simulink model "fusionAlg"  (R2018b)
settings: Solver=FixedStepDiscrete  StartTime=0.0  StopTime=inf  FixedStep=0.01  RelTol=1e-3
PostLoadFcn:
  | if any(exist('dsrtsu_mdlpostloadfcn', 'file') ~= 0), dsrtsu_mdlpostloadfcn('Execute', bdroot); end
model workspace (MAT data in the model file):
  handle : class17 (value not decoded)
(part 3 of 24)

== system fusionAlg/FUSION /FUS_DataAdapter/RadarAdapter/Subsystem42 ==
  <x6B_3B_Obj_27> : Inport
  Bus Creator : BusCreator  Inputs=2  OutDataTypeStr=Bus: FUS_UINT8_RESERVED_ST
      settings: InheritFromInputs=off
  Bus Creator1 : BusCreator  Inputs=17  OutDataTypeStr=Bus: FUS_RADAR_OBJ_ST  NonVirtualBus=on
      settings: InheritFromInputs=off
  Bus Selector1 : BusSelector  OutputSignals=Obj_ObstacleProb,Obj_XPos_Stdev,Obj_YPos_Stdev,Obj_XVelRel_Stdev,Obj_XAccRel,Obj_ExstProb,Obj_YVelRel,Obj_XVelRel,Obj_XPos,Obj_YPos,Obj_ID,Obj_UpdateFlag,Obj_ValidFlag,Obj_MotionPattern,Obj_Type,Obj_MeasFlag
  Constant : Constant  Value=0  OutDataTypeStr=uint8
  Constant1 : Constant  Value=0  OutDataTypeStr=uint8
  Data Type Conversion : DataTypeConversion  OutDataTypeStr=uint16
  Data Type Conversion{1..5} (5 alike) : DataTypeConversion  OutDataTypeStr=uint8
  <OBJ_27> : Outport
  wires:
  Bus Selector1/10 -> Bus Creator1/10  "<Obj_YPos>"
  Constant1/1 -> Bus Creator/2
  Bus Selector1/8 -> Bus Creator1/8  "<Obj_XVelRel>"
  Bus Selector1/14 -> Data Type Conversion3/1  "<Obj_MotionPattern>"
  Bus Creator1/1 -> <OBJ_27>/1
  Bus Selector1/11 -> Data Type Conversion/1  "<Obj_ID>"
  Bus Selector1/16 -> Data Type Conversion5/1  "<Obj_MeasFlag>"
  Bus Selector1/2 -> Bus Creator1/2  "<Obj_XPos_Stdev>"
  Bus Selector1/6 -> Bus Creator1/6  "<Obj_ExstProb>"
  Bus Selector1/1 -> Bus Creator1/1  "<Obj_ObstacleProb>"
  Bus Selector1/15 -> Data Type Conversion4/1  "<Obj_Type>"
  Constant/1 -> Bus Creator/1
  Bus Selector1/13 -> Data Type Conversion2/1  "<Obj_ValidFlag>"
  Bus Selector1/9 -> Bus Creator1/9  "<Obj_XPos>"
  Bus Selector1/4 -> Bus Creator1/4  "<Obj_XVelRel_Stdev>"
  Bus Selector1/3 -> Bus Creator1/3  "<Obj_YPos_Stdev>"
  Bus Selector1/5 -> Bus Creator1/5  "<Obj_XAccRel>"
  Bus Selector1/7 -> Bus Creator1/7  "<Obj_YVelRel>"
  Bus Selector1/12 -> Data Type Conversion1/1  "<Obj_UpdateFlag>"
  <x6B_3B_Obj_27>/1 -> Bus Selector1/1
  Bus Creator/1 -> Bus Creator1/17
  Data Type Conversion/1 -> Bus Creator1/11
  Data Type Conversion1/1 -> Bus Creator1/12
  Data Type Conversion2/1 -> Bus Creator1/13
  Data Type Conversion3/1 -> Bus Creator1/14
  Data Type Conversion4/1 -> Bus Creator1/15
  Data Type Conversion5/1 -> Bus Creator1/16

== system fusionAlg/FUSION /FUS_DataAdapter/RadarAdapter/Subsystem43 ==
  <x6C_3C_Obj_28> : Inport
  Bus Creator : BusCreator  Inputs=2  OutDataTypeStr=Bus: FUS_UINT8_RESERVED_ST
      settings: InheritFromInputs=off
  Bus Creator1 : BusCreator  Inputs=17  OutDataTypeStr=Bus: FUS_RADAR_OBJ_ST  NonVirtualBus=on
      settings: InheritFromInputs=off
  Bus Selector1 : BusSelector  OutputSignals=Obj_ObstacleProb,Obj_XPos_Stdev,Obj_YPos_Stdev,Obj_XVelRel_Stdev,Obj_XAccRel,Obj_ExstProb,Obj_YVelRel,Obj_XVelRel,Obj_XPos,Obj_YPos,Obj_ID,Obj_UpdateFlag,Obj_ValidFlag,Obj_MotionPattern,Obj_Type,Obj_MeasFlag
  Constant : Constant  Value=0  OutDataTypeStr=uint8
  Constant1 : Constant  Value=0  OutDataTypeStr=uint8
  Data Type Conversion : DataTypeConversion  OutDataTypeStr=uint16
  Data Type Conversion{1..5} (5 alike) : DataTypeConversion  OutDataTypeStr=uint8
  <OBJ_28> : Outport
  wires:
  Bus Selector1/10 -> Bus Creator1/10  "<Obj_YPos>"
  Constant1/1 -> Bus Creator/2
  Bus Selector1/8 -> Bus Creator1/8  "<Obj_XVelRel>"
  Bus Selector1/14 -> Data Type Conversion3/1  "<Obj_MotionPattern>"
  Bus Creator1/1 -> <OBJ_28>/1
  Bus Selector1/11 -> Data Type Conversion/1  "<Obj_ID>"
  Bus Selector1/16 -> Data Type Conversion5/1  "<Obj_MeasFlag>"
  Bus Selector1/2 -> Bus Creator1/2  "<Obj_XPos_Stdev>"
  Bus Selector1/6 -> Bus Creator1/6  "<Obj_ExstProb>"
  Bus Selector1/1 -> Bus Creator1/1  "<Obj_ObstacleProb>"
  Bus Selector1/15 -> Data Type Conversion4/1  "<Obj_Type>"
  Constant/1 -> Bus Creator/1
  Bus Selector1/13 -> Data Type Conversion2/1  "<Obj_ValidFlag>"
  Bus Selector1/9 -> Bus Creator1/9  "<Obj_XPos>"
  Bus Selector1/4 -> Bus Creator1/4  "<Obj_XVelRel_Stdev>"
  Bus Selector1/3 -> Bus Creator1/3  "<Obj_YPos_Stdev>"
  Bus Selector1/5 -> Bus Creator1/5  "<Obj_XAccRel>"
  Bus Selector1/7 -> Bus Creator1/7  "<Obj_YVelRel>"
  Bus Selector1/12 -> Data Type Conversion1/1  "<Obj_UpdateFlag>"
  <x6C_3C_Obj_28>/1 -> Bus Selector1/1
  Bus Creator/1 -> Bus Creator1/17
  Data Type Conversion/1 -> Bus Creator1/11
  Data Type Conversion1/1 -> Bus Creator1/12
  Data Type Conversion2/1 -> Bus Creator1/13
  Data Type Conversion3/1 -> Bus Creator1/14
  Data Type Conversion4/1 -> Bus Creator1/15
  Data Type Conversion5/1 -> Bus Creator1/16

== system fusionAlg/FUSION /FUS_DataAdapter/RadarAdapter/Subsystem44 ==
  <x6D_3D_Obj_29> : Inport
  Bus Creator : BusCreator  Inputs=2  OutDataTypeStr=Bus: FUS_UINT8_RESERVED_ST
      settings: InheritFromInputs=off
  Bus Creator1 : BusCreator  Inputs=17  OutDataTypeStr=Bus: FUS_RADAR_OBJ_ST  NonVirtualBus=on
      settings: InheritFromInputs=off
  Bus Selector1 : BusSelector  OutputSignals=Obj_ObstacleProb,Obj_XPos_Stdev,Obj_YPos_Stdev,Obj_XVelRel_Stdev,Obj_XAccRel,Obj_ExstProb,Obj_YVelRel,Obj_XVelRel,Obj_XPos,Obj_YPos,Obj_ID,Obj_UpdateFlag,Obj_ValidFlag,Obj_MotionPattern,Obj_Type,Obj_MeasFlag
  Constant : Constant  Value=0  OutDataTypeStr=uint8
  Constant1 : Constant  Value=0  OutDataTypeStr=uint8
  Data Type Conversion : DataTypeConversion  OutDataTypeStr=uint16
  Data Type Conversion{1..5} (5 alike) : DataTypeConversion  OutDataTypeStr=uint8
  <OBJ_29> : Outport
  wires:
  Bus Selector1/10 -> Bus Creator1/10  "<Obj_YPos>"
  Constant1/1 -> Bus Creator/2
  Bus Selector1/8 -> Bus Creator1/8  "<Obj_XVelRel>"
  Bus Selector1/14 -> Data Type Conversion3/1  "<Obj_MotionPattern>"
  Bus Creator1/1 -> <OBJ_29>/1
  Bus Selector1/11 -> Data Type Conversion/1  "<Obj_ID>"
  Bus Selector1/16 -> Data Type Conversion5/1  "<Obj_MeasFlag>"
  Bus Selector1/2 -> Bus Creator1/2  "<Obj_XPos_Stdev>"
  Bus Selector1/6 -> Bus Creator1/6  "<Obj_ExstProb>"
  Bus Selector1/1 -> Bus Creator1/1  "<Obj_ObstacleProb>"
  Bus Selector1/15 -> Data Type Conversion4/1  "<Obj_Type>"
  Constant/1 -> Bus Creator/1
  Bus Selector1/13 -> Data Type Conversion2/1  "<Obj_ValidFlag>"
  Bus Selector1/9 -> Bus Creator1/9  "<Obj_XPos>"
  Bus Selector1/4 -> Bus Creator1/4  "<Obj_XVelRel_Stdev>"
  Bus Selector1/3 -> Bus Creator1/3  "<Obj_YPos_Stdev>"
  Bus Selector1/5 -> Bus Creator1/5  "<Obj_XAccRel>"
  Bus Selector1/7 -> Bus Creator1/7  "<Obj_YVelRel>"
  Bus Selector1/12 -> Data Type Conversion1/1  "<Obj_UpdateFlag>"
  <x6D_3D_Obj_29>/1 -> Bus Selector1/1
  Bus Creator/1 -> Bus Creator1/17
  Data Type Conversion/1 -> Bus Creator1/11
  Data Type Conversion1/1 -> Bus Creator1/12
  Data Type Conversion2/1 -> Bus Creator1/13
  Data Type Conversion3/1 -> Bus Creator1/14
  Data Type Conversion4/1 -> Bus Creator1/15
  Data Type Conversion5/1 -> Bus Creator1/16

== system fusionAlg/FUSION /FUS_DataAdapter/RadarAdapter/Subsystem45 ==
  <x6E_3E_Obj_30> : Inport
  Bus Creator : BusCreator  Inputs=2  OutDataTypeStr=Bus: FUS_UINT8_RESERVED_ST
      settings: InheritFromInputs=off
  Bus Creator1 : BusCreator  Inputs=17  OutDataTypeStr=Bus: FUS_RADAR_OBJ_ST  NonVirtualBus=on
      settings: InheritFromInputs=off
  Bus Selector1 : BusSelector  OutputSignals=Obj_ObstacleProb,Obj_XPos_Stdev,Obj_YPos_Stdev,Obj_XVelRel_Stdev,Obj_XAccRel,Obj_ExstProb,Obj_YVelRel,Obj_XVelRel,Obj_XPos,Obj_YPos,Obj_ID,Obj_UpdateFlag,Obj_ValidFlag,Obj_MotionPattern,Obj_Type,Obj_MeasFlag
  Constant : Constant  Value=0  OutDataTypeStr=uint8
  Constant1 : Constant  Value=0  OutDataTypeStr=uint8
  Data Type Conversion : DataTypeConversion  OutDataTypeStr=uint16
  Data Type Conversion{1..5} (5 alike) : DataTypeConversion  OutDataTypeStr=uint8
  <OBJ_30> : Outport
  wires:
  Bus Selector1/10 -> Bus Creator1/10  "<Obj_YPos>"
  Constant1/1 -> Bus Creator/2
  Bus Selector1/8 -> Bus Creator1/8  "<Obj_XVelRel>"
  Bus Selector1/14 -> Data Type Conversion3/1  "<Obj_MotionPattern>"
  Bus Creator1/1 -> <OBJ_30>/1
  Bus Selector1/11 -> Data Type Conversion/1  "<Obj_ID>"
  Bus Selector1/16 -> Data Type Conversion5/1  "<Obj_MeasFlag>"
  Bus Selector1/2 -> Bus Creator1/2  "<Obj_XPos_Stdev>"
  Bus Selector1/6 -> Bus Creator1/6  "<Obj_ExstProb>"
  Bus Selector1/1 -> Bus Creator1/1  "<Obj_ObstacleProb>"
  Bus Selector1/15 -> Data Type Conversion4/1  "<Obj_Type>"
  Constant/1 -> Bus Creator/1
  Bus Selector1/13 -> Data Type Conversion2/1  "<Obj_ValidFlag>"
  Bus Selector1/9 -> Bus Creator1/9  "<Obj_XPos>"
  Bus Selector1/4 -> Bus Creator1/4  "<Obj_XVelRel_Stdev>"
  Bus Selector1/3 -> Bus Creator1/3  "<Obj_YPos_Stdev>"
  Bus Selector1/5 -> Bus Creator1/5  "<Obj_XAccRel>"
  Bus Selector1/7 -> Bus Creator1/7  "<Obj_YVelRel>"
  Bus Selector1/12 -> Data Type Conversion1/1  "<Obj_UpdateFlag>"
  <x6E_3E_Obj_30>/1 -> Bus Selector1/1
  Bus Creator/1 -> Bus Creator1/17
  Data Type Conversion/1 -> Bus Creator1/11
  Data Type Conversion1/1 -> Bus Creator1/12
  Data Type Conversion2/1 -> Bus Creator1/13
  Data Type Conversion3/1 -> Bus Creator1/14
  Data Type Conversion4/1 -> Bus Creator1/15
  Data Type Conversion5/1 -> Bus Creator1/16

== system fusionAlg/FUSION /FUS_DataAdapter/RadarAdapter/Subsystem46 ==
  <x6F_3F_Obj_31> : Inport
  Bus Creator : BusCreator  Inputs=2  OutDataTypeStr=Bus: FUS_UINT8_RESERVED_ST
      settings: InheritFromInputs=off
  Bus Creator1 : BusCreator  Inputs=17  OutDataTypeStr=Bus: FUS_RADAR_OBJ_ST  NonVirtualBus=on
      settings: InheritFromInputs=off
  Bus Selector1 : BusSelector  OutputSignals=Obj_ObstacleProb,Obj_XPos_Stdev,Obj_YPos_Stdev,Obj_XVelRel_Stdev,Obj_XAccRel,Obj_ExstProb,Obj_YVelRel,Obj_XVelRel,Obj_XPos,Obj_YPos,Obj_ID,Obj_UpdateFlag,Obj_ValidFlag,Obj_MotionPattern,Obj_Type,Obj_MeasFlag
  Constant : Constant  Value=0  OutDataTypeStr=uint8
  Constant1 : Constant  Value=0  OutDataTypeStr=uint8
  Data Type Conversion : DataTypeConversion  OutDataTypeStr=uint16
  Data Type Conversion{1..5} (5 alike) : DataTypeConversion  OutDataTypeStr=uint8
  <OBJ_31> : Outport
  wires:
  Bus Selector1/10 -> Bus Creator1/10  "<Obj_YPos>"
  Constant1/1 -> Bus Creator/2
  Bus Selector1/8 -> Bus Creator1/8  "<Obj_XVelRel>"
  Bus Selector1/14 -> Data Type Conversion3/1  "<Obj_MotionPattern>"
  Bus Creator1/1 -> <OBJ_31>/1
  Bus Selector1/11 -> Data Type Conversion/1  "<Obj_ID>"
  Bus Selector1/16 -> Data Type Conversion5/1  "<Obj_MeasFlag>"
  Bus Selector1/2 -> Bus Creator1/2  "<Obj_XPos_Stdev>"
  Bus Selector1/6 -> Bus Creator1/6  "<Obj_ExstProb>"
  Bus Selector1/1 -> Bus Creator1/1  "<Obj_ObstacleProb>"
  Bus Selector1/15 -> Data Type Conversion4/1  "<Obj_Type>"
  Constant/1 -> Bus Creator/1
  Bus Selector1/13 -> Data Type Conversion2/1  "<Obj_ValidFlag>"
  Bus Selector1/9 -> Bus Creator1/9  "<Obj_XPos>"
  Bus Selector1/4 -> Bus Creator1/4  "<Obj_XVelRel_Stdev>"
  Bus Selector1/3 -> Bus Creator1/3  "<Obj_YPos_Stdev>"
  Bus Selector1/5 -> Bus Creator1/5  "<Obj_XAccRel>"
  Bus Selector1/7 -> Bus Creator1/7  "<Obj_YVelRel>"
  Bus Selector1/12 -> Data Type Conversion1/1  "<Obj_UpdateFlag>"
  <x6F_3F_Obj_31>/1 -> Bus Selector1/1
  Bus Creator/1 -> Bus Creator1/17
  Data Type Conversion/1 -> Bus Creator1/11
  Data Type Conversion1/1 -> Bus Creator1/12
  Data Type Conversion2/1 -> Bus Creator1/13
  Data Type Conversion3/1 -> Bus Creator1/14
  Data Type Conversion4/1 -> Bus Creator1/15
  Data Type Conversion5/1 -> Bus Creator1/16

== system fusionAlg/FUSION /FUS_DataAdapter/RadarAdapter/Subsystem47 ==
  <x70_40_Obj_32> : Inport
  Bus Creator : BusCreator  Inputs=2  OutDataTypeStr=Bus: FUS_UINT8_RESERVED_ST
      settings: InheritFromInputs=off
  Bus Creator1 : BusCreator  Inputs=17  OutDataTypeStr=Bus: FUS_RADAR_OBJ_ST  NonVirtualBus=on
      settings: InheritFromInputs=off
  Bus Selector1 : BusSelector  OutputSignals=Obj_ObstacleProb,Obj_XPos_Stdev,Obj_YPos_Stdev,Obj_XVelRel_Stdev,Obj_XAccRel,Obj_ExstProb,Obj_YVelRel,Obj_XVelRel,Obj_XPos,Obj_YPos,Obj_ID,Obj_UpdateFlag,Obj_ValidFlag,Obj_MotionPattern,Obj_Type,Obj_MeasFlag
  Constant : Constant  Value=0  OutDataTypeStr=uint8
  Constant1 : Constant  Value=0  OutDataTypeStr=uint8
  Data Type Conversion : DataTypeConversion  OutDataTypeStr=uint16
  Data Type Conversion{1..5} (5 alike) : DataTypeConversion  OutDataTypeStr=uint8
  <OBJ_32> : Outport
  wires:
  Bus Selector1/10 -> Bus Creator1/10  "<Obj_YPos>"
  Constant1/1 -> Bus Creator/2
  Bus Selector1/8 -> Bus Creator1/8  "<Obj_XVelRel>"
  Bus Selector1/14 -> Data Type Conversion3/1  "<Obj_MotionPattern>"
  Bus Creator1/1 -> <OBJ_32>/1
  Bus Selector1/11 -> Data Type Conversion/1  "<Obj_ID>"
  Bus Selector1/16 -> Data Type Conversion5/1  "<Obj_MeasFlag>"
  Bus Selector1/2 -> Bus Creator1/2  "<Obj_XPos_Stdev>"
  Bus Selector1/6 -> Bus Creator1/6  "<Obj_ExstProb>"
  Bus Selector1/1 -> Bus Creator1/1  "<Obj_ObstacleProb>"
  Bus Selector1/15 -> Data Type Conversion4/1  "<Obj_Type>"
  Constant/1 -> Bus Creator/1
  Bus Selector1/13 -> Data Type Conversion2/1  "<Obj_ValidFlag>"
  Bus Selector1/9 -> Bus Creator1/9  "<Obj_XPos>"
  Bus Selector1/4 -> Bus Creator1/4  "<Obj_XVelRel_Stdev>"
  Bus Selector1/3 -> Bus Creator1/3  "<Obj_YPos_Stdev>"
  Bus Selector1/5 -> Bus Creator1/5  "<Obj_XAccRel>"
  Bus Selector1/7 -> Bus Creator1/7  "<Obj_YVelRel>"
  Bus Selector1/12 -> Data Type Conversion1/1  "<Obj_UpdateFlag>"
  <x70_40_Obj_32>/1 -> Bus Selector1/1
  Bus Creator/1 -> Bus Creator1/17
  Data Type Conversion/1 -> Bus Creator1/11
  Data Type Conversion1/1 -> Bus Creator1/12
  Data Type Conversion2/1 -> Bus Creator1/13
  Data Type Conversion3/1 -> Bus Creator1/14
  Data Type Conversion4/1 -> Bus Creator1/15
  Data Type Conversion5/1 -> Bus Creator1/16

== system fusionAlg/FUSION /FUS_DataAdapter/RadarAdapter/Subsystem48 ==
  <x71_41_Obj_33> : Inport
  Bus Creator : BusCreator  Inputs=2  OutDataTypeStr=Bus: FUS_UINT8_RESERVED_ST
      settings: InheritFromInputs=off
  Bus Creator1 : BusCreator  Inputs=17  OutDataTypeStr=Bus: FUS_RADAR_OBJ_ST  NonVirtualBus=on
      settings: InheritFromInputs=off
  Bus Selector1 : BusSelector  OutputSignals=Obj_ObstacleProb,Obj_XPos_Stdev,Obj_YPos_Stdev,Obj_XVelRel_Stdev,Obj_XAccRel,Obj_ExstProb,Obj_YVelRel,Obj_XVelRel,Obj_XPos,Obj_YPos,Obj_ID,Obj_UpdateFlag,Obj_ValidFlag,Obj_MotionPattern,Obj_Type,Obj_MeasFlag
  Constant : Constant  Value=0  OutDataTypeStr=uint8
  Constant1 : Constant  Value=0  OutDataTypeStr=uint8
  Data Type Conversion : DataTypeConversion  OutDataTypeStr=uint16
  Data Type Conversion{1..5} (5 alike) : DataTypeConversion  OutDataTypeStr=uint8
  <OBJ_33> : Outport
  wires:
  Bus Selector1/10 -> Bus Creator1/10  "<Obj_YPos>"
  Constant1/1 -> Bus Creator/2
  Bus Selector1/8 -> Bus Creator1/8  "<Obj_XVelRel>"
  Bus Selector1/14 -> Data Type Conversion3/1  "<Obj_MotionPattern>"
  Bus Creator1/1 -> <OBJ_33>/1
  Bus Selector1/11 -> Data Type Conversion/1  "<Obj_ID>"
  Bus Selector1/16 -> Data Type Conversion5/1  "<Obj_MeasFlag>"
  Bus Selector1/2 -> Bus Creator1/2  "<Obj_XPos_Stdev>"
  Bus Selector1/6 -> Bus Creator1/6  "<Obj_ExstProb>"
  Bus Selector1/1 -> Bus Creator1/1  "<Obj_ObstacleProb>"
  Bus Selector1/15 -> Data Type Conversion4/1  "<Obj_Type>"
  Constant/1 -> Bus Creator/1
  Bus Selector1/13 -> Data Type Conversion2/1  "<Obj_ValidFlag>"
  Bus Selector1/9 -> Bus Creator1/9  "<Obj_XPos>"
  Bus Selector1/4 -> Bus Creator1/4  "<Obj_XVelRel_Stdev>"
  Bus Selector1/3 -> Bus Creator1/3  "<Obj_YPos_Stdev>"
  Bus Selector1/5 -> Bus Creator1/5  "<Obj_XAccRel>"
  Bus Selector1/7 -> Bus Creator1/7  "<Obj_YVelRel>"
  Bus Selector1/12 -> Data Type Conversion1/1  "<Obj_UpdateFlag>"
  <x71_41_Obj_33>/1 -> Bus Selector1/1
  Bus Creator/1 -> Bus Creator1/17
  Data Type Conversion/1 -> Bus Creator1/11
  Data Type Conversion1/1 -> Bus Creator1/12
  Data Type Conversion2/1 -> Bus Creator1/13
  Data Type Conversion3/1 -> Bus Creator1/14
  Data Type Conversion4/1 -> Bus Creator1/15
  Data Type Conversion5/1 -> Bus Creator1/16

== system fusionAlg/FUSION /FUS_DataAdapter/RadarAdapter/Subsystem5 ==
  <x55_25_Obj_05> : Inport
  Bus Creator : BusCreator  Inputs=2  OutDataTypeStr=Bus: FUS_UINT8_RESERVED_ST
      settings: InheritFromInputs=off
  Bus Creator1 : BusCreator  Inputs=17  OutDataTypeStr=Bus: FUS_RADAR_OBJ_ST  NonVirtualBus=on
      settings: InheritFromInputs=off
  Bus Selector1 : BusSelector  OutputSignals=Obj_ObstacleProb,Obj_XPos_Stdev,Obj_YPos_Stdev,Obj_XVelRel_Stdev,Obj_XAccRel,Obj_ExstProb,Obj_YVelRel,Obj_XVelRel,Obj_XPos,Obj_YPos,Obj_ID,Obj_UpdateFlag,Obj_ValidFlag,Obj_MotionPattern,Obj_Type,Obj_MeasFlag
  Constant : Constant  Value=0  OutDataTypeStr=uint8
  Constant1 : Constant  Value=0  OutDataTypeStr=uint8
  Data Type Conversion : DataTypeConversion  OutDataTypeStr=uint16
  Data Type Conversion{1..5} (5 alike) : DataTypeConversion  OutDataTypeStr=uint8
  <OBJ_05> : Outport
  wires:
  Bus Selector1/10 -> Bus Creator1/10  "<Obj_YPos>"
  Constant1/1 -> Bus Creator/2
  Bus Selector1/8 -> Bus Creator1/8  "<Obj_XVelRel>"
  Bus Selector1/14 -> Data Type Conversion3/1  "<Obj_MotionPattern>"
  Bus Creator1/1 -> <OBJ_05>/1
  Bus Selector1/11 -> Data Type Conversion/1  "<Obj_ID>"
  Bus Selector1/16 -> Data Type Conversion5/1  "<Obj_MeasFlag>"
  Bus Selector1/2 -> Bus Creator1/2  "<Obj_XPos_Stdev>"
  Bus Selector1/6 -> Bus Creator1/6  "<Obj_ExstProb>"
  Bus Selector1/1 -> Bus Creator1/1  "<Obj_ObstacleProb>"
  Bus Selector1/15 -> Data Type Conversion4/1  "<Obj_Type>"
  Constant/1 -> Bus Creator/1
  Bus Selector1/13 -> Data Type Conversion2/1  "<Obj_ValidFlag>"
  Bus Selector1/9 -> Bus Creator1/9  "<Obj_XPos>"
  Bus Selector1/4 -> Bus Creator1/4  "<Obj_XVelRel_Stdev>"
  Bus Selector1/3 -> Bus Creator1/3  "<Obj_YPos_Stdev>"
  Bus Selector1/5 -> Bus Creator1/5  "<Obj_XAccRel>"
  Bus Selector1/7 -> Bus Creator1/7  "<Obj_YVelRel>"
  Bus Selector1/12 -> Data Type Conversion1/1  "<Obj_UpdateFlag>"
  <x55_25_Obj_05>/1 -> Bus Selector1/1
  Bus Creator/1 -> Bus Creator1/17
  Data Type Conversion/1 -> Bus Creator1/11
  Data Type Conversion1/1 -> Bus Creator1/12
  Data Type Conversion2/1 -> Bus Creator1/13
  Data Type Conversion3/1 -> Bus Creator1/14
  Data Type Conversion4/1 -> Bus Creator1/15
  Data Type Conversion5/1 -> Bus Creator1/16

== system fusionAlg/FUSION /FUS_DataAdapter/RadarAdapter/Subsystem6 ==
  <x56_26_Obj_06> : Inport
  Bus Creator : BusCreator  Inputs=2  OutDataTypeStr=Bus: FUS_UINT8_RESERVED_ST
      settings: InheritFromInputs=off
  Bus Creator1 : BusCreator  Inputs=17  OutDataTypeStr=Bus: FUS_RADAR_OBJ_ST  NonVirtualBus=on
      settings: InheritFromInputs=off
  Bus Selector1 : BusSelector  OutputSignals=Obj_ObstacleProb,Obj_XPos_Stdev,Obj_YPos_Stdev,Obj_XVelRel_Stdev,Obj_XAccRel,Obj_ExstProb,Obj_YVelRel,Obj_XVelRel,Obj_XPos,Obj_YPos,Obj_ID,Obj_UpdateFlag,Obj_ValidFlag,Obj_MotionPattern,Obj_Type,Obj_MeasFlag
  Constant : Constant  Value=0  OutDataTypeStr=uint8
  Constant1 : Constant  Value=0  OutDataTypeStr=uint8
  Data Type Conversion : DataTypeConversion  OutDataTypeStr=uint16
  Data Type Conversion{1..5} (5 alike) : DataTypeConversion  OutDataTypeStr=uint8
  <OBJ_06> : Outport
  wires:
  Bus Selector1/10 -> Bus Creator1/10  "<Obj_YPos>"
  Constant1/1 -> Bus Creator/2
  Bus Selector1/8 -> Bus Creator1/8  "<Obj_XVelRel>"
  Bus Selector1/14 -> Data Type Conversion3/1  "<Obj_MotionPattern>"
  Bus Creator1/1 -> <OBJ_06>/1
  Bus Selector1/11 -> Data Type Conversion/1  "<Obj_ID>"
  Bus Selector1/16 -> Data Type Conversion5/1  "<Obj_MeasFlag>"
  Bus Selector1/2 -> Bus Creator1/2  "<Obj_XPos_Stdev>"
  Bus Selector1/6 -> Bus Creator1/6  "<Obj_ExstProb>"
  Bus Selector1/1 -> Bus Creator1/1  "<Obj_ObstacleProb>"
  Bus Selector1/15 -> Data Type Conversion4/1  "<Obj_Type>"
  Constant/1 -> Bus Creator/1
  Bus Selector1/13 -> Data Type Conversion2/1  "<Obj_ValidFlag>"
  Bus Selector1/9 -> Bus Creator1/9  "<Obj_XPos>"
  Bus Selector1/4 -> Bus Creator1/4  "<Obj_XVelRel_Stdev>"
  Bus Selector1/3 -> Bus Creator1/3  "<Obj_YPos_Stdev>"
  Bus Selector1/5 -> Bus Creator1/5  "<Obj_XAccRel>"
  Bus Selector1/7 -> Bus Creator1/7  "<Obj_YVelRel>"
  Bus Selector1/12 -> Data Type Conversion1/1  "<Obj_UpdateFlag>"
  <x56_26_Obj_06>/1 -> Bus Selector1/1
  Bus Creator/1 -> Bus Creator1/17
  Data Type Conversion/1 -> Bus Creator1/11
  Data Type Conversion1/1 -> Bus Creator1/12
  Data Type Conversion2/1 -> Bus Creator1/13
  Data Type Conversion3/1 -> Bus Creator1/14
  Data Type Conversion4/1 -> Bus Creator1/15
  Data Type Conversion5/1 -> Bus Creator1/16

== system fusionAlg/FUSION /FUS_DataAdapter/RadarAdapter/Subsystem7 ==
  <x57_27_Obj_07> : Inport
  Bus Creator : BusCreator  Inputs=2  OutDataTypeStr=Bus: FUS_UINT8_RESERVED_ST
      settings: InheritFromInputs=off
  Bus Creator1 : BusCreator  Inputs=17  OutDataTypeStr=Bus: FUS_RADAR_OBJ_ST  NonVirtualBus=on
      settings: InheritFromInputs=off
  Bus Selector1 : BusSelector  OutputSignals=Obj_ObstacleProb,Obj_XPos_Stdev,Obj_YPos_Stdev,Obj_XVelRel_Stdev,Obj_XAccRel,Obj_ExstProb,Obj_YVelRel,Obj_XVelRel,Obj_XPos,Obj_YPos,Obj_ID,Obj_UpdateFlag,Obj_ValidFlag,Obj_MotionPattern,Obj_Type,Obj_MeasFlag
  Constant : Constant  Value=0  OutDataTypeStr=uint8
  Constant1 : Constant  Value=0  OutDataTypeStr=uint8
  Data Type Conversion : DataTypeConversion  OutDataTypeStr=uint16
  Data Type Conversion{1..5} (5 alike) : DataTypeConversion  OutDataTypeStr=uint8
  <OBJ_07> : Outport
  wires:
  Bus Selector1/10 -> Bus Creator1/10  "<Obj_YPos>"
  Constant1/1 -> Bus Creator/2
  Bus Selector1/8 -> Bus Creator1/8  "<Obj_XVelRel>"
  Bus Selector1/14 -> Data Type Conversion3/1  "<Obj_MotionPattern>"
  Bus Creator1/1 -> <OBJ_07>/1
  Bus Selector1/11 -> Data Type Conversion/1  "<Obj_ID>"
  Bus Selector1/16 -> Data Type Conversion5/1  "<Obj_MeasFlag>"
  Bus Selector1/2 -> Bus Creator1/2  "<Obj_XPos_Stdev>"
  Bus Selector1/6 -> Bus Creator1/6  "<Obj_ExstProb>"
  Bus Selector1/1 -> Bus Creator1/1  "<Obj_ObstacleProb>"
  Bus Selector1/15 -> Data Type Conversion4/1  "<Obj_Type>"
  Constant/1 -> Bus Creator/1
  Bus Selector1/13 -> Data Type Conversion2/1  "<Obj_ValidFlag>"
  Bus Selector1/9 -> Bus Creator1/9  "<Obj_XPos>"
  Bus Selector1/4 -> Bus Creator1/4  "<Obj_XVelRel_Stdev>"
  Bus Selector1/3 -> Bus Creator1/3  "<Obj_YPos_Stdev>"
  Bus Selector1/5 -> Bus Creator1/5  "<Obj_XAccRel>"
  Bus Selector1/7 -> Bus Creator1/7  "<Obj_YVelRel>"
  Bus Selector1/12 -> Data Type Conversion1/1  "<Obj_UpdateFlag>"
  <x57_27_Obj_07>/1 -> Bus Selector1/1
  Bus Creator/1 -> Bus Creator1/17
  Data Type Conversion/1 -> Bus Creator1/11
  Data Type Conversion1/1 -> Bus Creator1/12
  Data Type Conversion2/1 -> Bus Creator1/13
  Data Type Conversion3/1 -> Bus Creator1/14
  Data Type Conversion4/1 -> Bus Creator1/15
  Data Type Conversion5/1 -> Bus Creator1/16

== system fusionAlg/FUSION /FUS_DataAdapter/RadarAdapter/Subsystem8 ==
  <x58_28_Obj_08> : Inport
  Bus Creator : BusCreator  Inputs=2  OutDataTypeStr=Bus: FUS_UINT8_RESERVED_ST
      settings: InheritFromInputs=off
  Bus Creator1 : BusCreator  Inputs=17  OutDataTypeStr=Bus: FUS_RADAR_OBJ_ST  NonVirtualBus=on
      settings: InheritFromInputs=off
  Bus Selector1 : BusSelector  OutputSignals=Obj_ObstacleProb,Obj_XPos_Stdev,Obj_YPos_Stdev,Obj_XVelRel_Stdev,Obj_XAccRel,Obj_ExstProb,Obj_YVelRel,Obj_XVelRel,Obj_XPos,Obj_YPos,Obj_ID,Obj_UpdateFlag,Obj_ValidFlag,Obj_MotionPattern,Obj_Type,Obj_MeasFlag
  Constant : Constant  Value=0  OutDataTypeStr=uint8
  Constant1 : Constant  Value=0  OutDataTypeStr=uint8
  Data Type Conversion : DataTypeConversion  OutDataTypeStr=uint16
  Data Type Conversion{1..5} (5 alike) : DataTypeConversion  OutDataTypeStr=uint8
  <OBJ_08> : Outport
  wires:
  Bus Selector1/10 -> Bus Creator1/10  "<Obj_YPos>"
  Constant1/1 -> Bus Creator/2
  Bus Selector1/8 -> Bus Creator1/8  "<Obj_XVelRel>"
  Bus Selector1/14 -> Data Type Conversion3/1  "<Obj_MotionPattern>"
  Bus Creator1/1 -> <OBJ_08>/1
  Bus Selector1/11 -> Data Type Conversion/1  "<Obj_ID>"
  Bus Selector1/16 -> Data Type Conversion5/1  "<Obj_MeasFlag>"
  Bus Selector1/2 -> Bus Creator1/2  "<Obj_XPos_Stdev>"
  Bus Selector1/6 -> Bus Creator1/6  "<Obj_ExstProb>"
  Bus Selector1/1 -> Bus Creator1/1  "<Obj_ObstacleProb>"
  Bus Selector1/15 -> Data Type Conversion4/1  "<Obj_Type>"
  Constant/1 -> Bus Creator/1
  Bus Selector1/13 -> Data Type Conversion2/1  "<Obj_ValidFlag>"
  Bus Selector1/9 -> Bus Creator1/9  "<Obj_XPos>"
  Bus Selector1/4 -> Bus Creator1/4  "<Obj_XVelRel_Stdev>"
  Bus Selector1/3 -> Bus Creator1/3  "<Obj_YPos_Stdev>"
  Bus Selector1/5 -> Bus Creator1/5  "<Obj_XAccRel>"
  Bus Selector1/7 -> Bus Creator1/7  "<Obj_YVelRel>"
  Bus Selector1/12 -> Data Type Conversion1/1  "<Obj_UpdateFlag>"
  <x58_28_Obj_08>/1 -> Bus Selector1/1
  Bus Creator/1 -> Bus Creator1/17
  Data Type Conversion/1 -> Bus Creator1/11
  Data Type Conversion1/1 -> Bus Creator1/12
  Data Type Conversion2/1 -> Bus Creator1/13
  Data Type Conversion3/1 -> Bus Creator1/14
  Data Type Conversion4/1 -> Bus Creator1/15
  Data Type Conversion5/1 -> Bus Creator1/16

== system fusionAlg/FUSION /FUS_DataAdapter/RadarAdapter/Subsystem9 ==
  <x59_29_Obj_09> : Inport
  Bus Creator : BusCreator  Inputs=2  OutDataTypeStr=Bus: FUS_UINT8_RESERVED_ST
      settings: InheritFromInputs=off
  Bus Creator1 : BusCreator  Inputs=17  OutDataTypeStr=Bus: FUS_RADAR_OBJ_ST  NonVirtualBus=on
      settings: InheritFromInputs=off
  Bus Selector1 : BusSelector  OutputSignals=Obj_ObstacleProb,Obj_XPos_Stdev,Obj_YPos_Stdev,Obj_XVelRel_Stdev,Obj_XAccRel,Obj_ExstProb,Obj_YVelRel,Obj_XVelRel,Obj_XPos,Obj_YPos,Obj_ID,Obj_UpdateFlag,Obj_ValidFlag,Obj_MotionPattern,Obj_Type,Obj_MeasFlag
  Constant : Constant  Value=0  OutDataTypeStr=uint8
  Constant1 : Constant  Value=0  OutDataTypeStr=uint8
  Data Type Conversion : DataTypeConversion  OutDataTypeStr=uint16
  Data Type Conversion{1..5} (5 alike) : DataTypeConversion  OutDataTypeStr=uint8
  <OBJ_09> : Outport
  wires:
  Bus Selector1/10 -> Bus Creator1/10  "<Obj_YPos>"
  Constant1/1 -> Bus Creator/2
  Bus Selector1/8 -> Bus Creator1/8  "<Obj_XVelRel>"
  Bus Selector1/14 -> Data Type Conversion3/1  "<Obj_MotionPattern>"
  Bus Creator1/1 -> <OBJ_09>/1
  Bus Selector1/11 -> Data Type Conversion/1  "<Obj_ID>"
  Bus Selector1/16 -> Data Type Conversion5/1  "<Obj_MeasFlag>"
  Bus Selector1/2 -> Bus Creator1/2  "<Obj_XPos_Stdev>"
  Bus Selector1/6 -> Bus Creator1/6  "<Obj_ExstProb>"
  Bus Selector1/1 -> Bus Creator1/1  "<Obj_ObstacleProb>"
  Bus Selector1/15 -> Data Type Conversion4/1  "<Obj_Type>"
  Constant/1 -> Bus Creator/1
  Bus Selector1/13 -> Data Type Conversion2/1  "<Obj_ValidFlag>"
  Bus Selector1/9 -> Bus Creator1/9  "<Obj_XPos>"
  Bus Selector1/4 -> Bus Creator1/4  "<Obj_XVelRel_Stdev>"
  Bus Selector1/3 -> Bus Creator1/3  "<Obj_YPos_Stdev>"
  Bus Selector1/5 -> Bus Creator1/5  "<Obj_XAccRel>"
  Bus Selector1/7 -> Bus Creator1/7  "<Obj_YVelRel>"
  Bus Selector1/12 -> Data Type Conversion1/1  "<Obj_UpdateFlag>"
  <x59_29_Obj_09>/1 -> Bus Selector1/1
  Bus Creator/1 -> Bus Creator1/17
  Data Type Conversion/1 -> Bus Creator1/11
  Data Type Conversion1/1 -> Bus Creator1/12
  Data Type Conversion2/1 -> Bus Creator1/13
  Data Type Conversion3/1 -> Bus Creator1/14
  Data Type Conversion4/1 -> Bus Creator1/15
  Data Type Conversion5/1 -> Bus Creator1/16

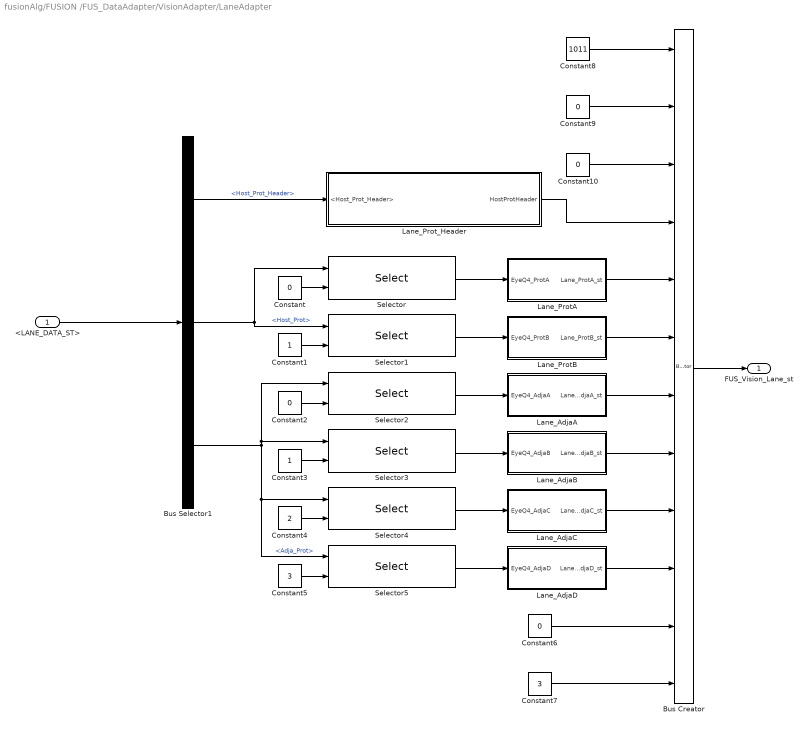
== system fusionAlg/FUSION /FUS_DataAdapter/VisionAdapter/LaneAdapter ==
  <LANE_DATA_ST> : Inport
  Bus Creator : BusCreator  Inputs=12  OutDataTypeStr=Bus: FUS_EYEQ4_LANE_DATA_ST  NonVirtualBus=on
      settings: InheritFromInputs=off
  Bus Selector1 : BusSelector  OutputSignals=Host_Prot_Header,Host_Prot,Adja_Prot
  Constant : Constant  Value=0  OutDataTypeStr=uint8
  Constant1 : Constant  OutDataTypeStr=uint8
  Constant10 : Constant  Value=0  OutDataTypeStr=uint32
  Constant2 : Constant  Value=0  OutDataTypeStr=uint8
  Constant3 : Constant  OutDataTypeStr=uint8
  Constant4 : Constant  Value=2  OutDataTypeStr=uint8
  Constant5 : Constant  Value=3  OutDataTypeStr=uint8
  Constant6 : Constant  Value=0  OutDataTypeStr=uint32
  Constant7 : Constant  Value=3  OutDataTypeStr=uint32
  Constant8 : Constant  Value=1011  OutDataTypeStr=double
  Constant9 : Constant  Value=0  OutDataTypeStr=uint32
  Lane_AdjaA : Subsystem
  Lane_AdjaB : Subsystem
  Lane_AdjaC : Subsystem
  Lane_AdjaD : Subsystem
  Lane_ProtA : Subsystem
  Lane_ProtB : Subsystem
  Lane_Prot_Header : Subsystem
  Selector : Selector  IndexMode=Zero-based  InputPortWidth=2  IndexOptions=Index vector (port)  Indices=[1 3]  OutputSizes=1
  Selector1 : Selector  IndexMode=Zero-based  InputPortWidth=2  IndexOptions=Index vector (port)  Indices=[1 3]  OutputSizes=1
  Selector{2..5} (4 alike) : Selector  IndexMode=Zero-based  InputPortWidth=4  IndexOptions=Index vector (port)  Indices=[1 3]  OutputSizes=1
  FUS_Vision_Lane_st : Outport  OutDataTypeStr=Bus: FUS_EYEQ4_LANE_DATA_ST
  wires:
  Bus Selector1/3 -> Selector2/1, Selector3/1, Selector5/1, Selector4/1  "<Adja_Prot>"
  <LANE_DATA_ST>/1 -> Bus Selector1/1
  Bus Creator/1 -> FUS_Vision_Lane_st/1
  Constant/1 -> Selector/2
  Bus Selector1/2 -> Selector/1, Selector1/1  "<Host_Prot>"
  Constant1/1 -> Selector1/2
  Selector1/1 -> Lane_ProtB/1(EyeQ4_ProtB)
  Constant2/1 -> Selector2/2
  Selector2/1 -> Lane_AdjaA/1(EyeQ4_AdjaA)
  Selector3/1 -> Lane_AdjaB/1(EyeQ4_AdjaB)
  Selector4/1 -> Lane_AdjaC/1(EyeQ4_AdjaC)
  Selector5/1 -> Lane_AdjaD/1(EyeQ4_AdjaD)
  Constant3/1 -> Selector3/2
  Constant4/1 -> Selector4/2
  Constant5/1 -> Selector5/2
  Constant6/1 -> Bus Creator/11
  Constant7/1 -> Bus Creator/12
  Constant8/1 -> Bus Creator/1
  Constant9/1 -> Bus Creator/2
  Constant10/1 -> Bus Creator/3
  Selector/1 -> Lane_ProtA/1(EyeQ4_ProtA)
  Lane_ProtA/1(Lane_ProtA_st) -> Bus Creator/5
  Lane_ProtB/1(Lane_ProtB_st) -> Bus Creator/6
  Lane_AdjaA/1(Lane_AdjaA_st) -> Bus Creator/7
  Lane_AdjaB/1(Lane_AdjaB_st) -> Bus Creator/8
  Lane_AdjaC/1(Lane_AdjaC_st) -> Bus Creator/9
  Lane_AdjaD/1(Lane_AdjaD_st) -> Bus Creator/10
  Bus Selector1/1 -> Lane_Prot_Header/1(<Host_Prot_Header>)  "<Host_Prot_Header>"
  Lane_Prot_Header/1(HostProtHeader) -> Bus Creator/4

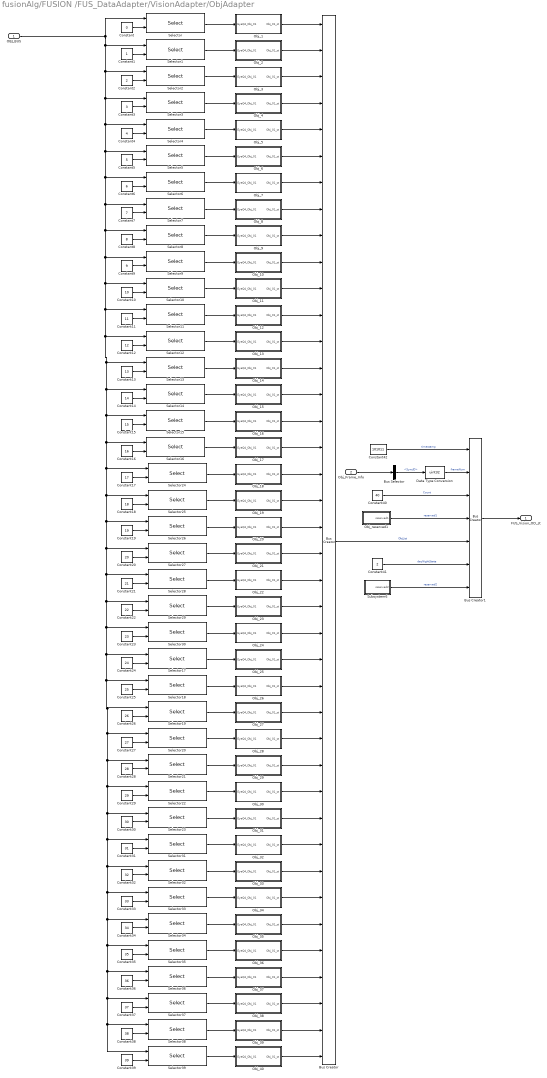
== system fusionAlg/FUSION /FUS_DataAdapter/VisionAdapter/ObjAdapter ==
  OBJ_BUS : Inport  OutDataTypeStr=Bus: OBJECT_ST
  Obj_Frame_Info : Inport  Port=2  OutDataTypeStr=Bus: OBJECT_FRAME_INFO
  Bus Creator : BusCreator  Inputs=40  OutDataTypeStr=Bus: FUS_VISION_OBJ_LIST_ST  NonVirtualBus=on
      settings: InheritFromInputs=off
  Bus Creator1 : BusCreator  Inputs=7  OutDataTypeStr=Bus: FUS_VISION_OBJ_DATA_ST  NonVirtualBus=on
      settings: InheritFromInputs=off
  Bus Selector : BusSelector  OutputSignals=SyncID
  Constant : Constant  Value=0  OutDataTypeStr=uint8
  Constant1 : Constant  OutDataTypeStr=uint8
  Constant10 : Constant  Value=10  OutDataTypeStr=uint8
  Constant11 : Constant  Value=11  OutDataTypeStr=uint8
  Constant12 : Constant  Value=12  OutDataTypeStr=uint8
  Constant13 : Constant  Value=13  OutDataTypeStr=uint8
  Constant14 : Constant  Value=14  OutDataTypeStr=uint8
  Constant15 : Constant  Value=15  OutDataTypeStr=uint8
  Constant16 : Constant  Value=16  OutDataTypeStr=uint8
  Constant17 : Constant  Value=17  OutDataTypeStr=uint8
  Constant18 : Constant  Value=18  OutDataTypeStr=uint8
  Constant19 : Constant  Value=19  OutDataTypeStr=uint8
  Constant2 : Constant  Value=2  OutDataTypeStr=uint8
  Constant20 : Constant  Value=20  OutDataTypeStr=uint8
  Constant21 : Constant  Value=21  OutDataTypeStr=uint8
  Constant22 : Constant  Value=22  OutDataTypeStr=uint8
  Constant23 : Constant  Value=23  OutDataTypeStr=uint8
  Constant24 : Constant  Value=24  OutDataTypeStr=uint8
  Constant25 : Constant  Value=25  OutDataTypeStr=uint8
  Constant26 : Constant  Value=26  OutDataTypeStr=uint8
  Constant27 : Constant  Value=27  OutDataTypeStr=uint8
  Constant28 : Constant  Value=28  OutDataTypeStr=uint8
  Constant29 : Constant  Value=29  OutDataTypeStr=uint8
  Constant3 : Constant  Value=3  OutDataTypeStr=uint8
  Constant30 : Constant  Value=30  OutDataTypeStr=uint8
  Constant31 : Constant  Value=31  OutDataTypeStr=uint8
  Constant32 : Constant  Value=32  OutDataTypeStr=uint8
  Constant33 : Constant  Value=33  OutDataTypeStr=uint8
  Constant34 : Constant  Value=34  OutDataTypeStr=uint8
  Constant35 : Constant  Value=35  OutDataTypeStr=uint8
  Constant36 : Constant  Value=36  OutDataTypeStr=uint8
  Constant37 : Constant  Value=37  OutDataTypeStr=uint8
  Constant38 : Constant  Value=38  OutDataTypeStr=uint8
  Constant39 : Constant  Value=39  OutDataTypeStr=uint8
  Constant4 : Constant  Value=4  OutDataTypeStr=uint8
  Constant40 : Constant  Value=40  OutDataTypeStr=uint8
  Constant41 : Constant  Value=2  OutDataTypeStr=uint32
  Constant42 : Constant  Value=101011  OutDataTypeStr=double
  Constant5 : Constant  Value=5  OutDataTypeStr=uint8
  Constant6 : Constant  Value=6  OutDataTypeStr=uint8
  Constant7 : Constant  Value=7  OutDataTypeStr=uint8
  Constant8 : Constant  Value=8  OutDataTypeStr=uint8
  Constant9 : Constant  Value=9  OutDataTypeStr=uint8
  Data Type Conversion : DataTypeConversion  OutDataTypeStr=uint32
  Obj_1 : Subsystem
  Obj_10 : Subsystem
  Obj_11 : Subsystem
  Obj_12 : Subsystem
  Obj_13 : Subsystem
  Obj_14 : Subsystem
  Obj_15 : Subsystem
  Obj_16 : Subsystem
  Obj_17 : Subsystem
  Obj_18 : Subsystem
  Obj_19 : Subsystem
  Obj_2 : Subsystem
  Obj_20 : Subsystem
  Obj_21 : Subsystem
  Obj_22 : Subsystem
  Obj_23 : Subsystem
  Obj_24 : Subsystem
  Obj_25 : Subsystem
  Obj_26 : Subsystem
  Obj_27 : Subsystem
  Obj_28 : Subsystem
  Obj_29 : Subsystem
  Obj_3 : Subsystem
  Obj_30 : Subsystem
  Obj_31 : Subsystem
  Obj_32 : Subsystem
  Obj_33 : Subsystem
  Obj_34 : Subsystem
  Obj_35 : Subsystem
  Obj_36 : Subsystem
  Obj_37 : Subsystem
  Obj_38 : Subsystem
  Obj_39 : Subsystem
  Obj_4 : Subsystem
  Obj_40 : Subsystem
  Obj_5 : Subsystem
  Obj_6 : Subsystem
  Obj_7 : Subsystem
  Obj_8 : Subsystem
  Obj_9 : Subsystem
  Obj_reserved1 : Subsystem
  Selector{,1..39} (40 alike) : Selector  IndexMode=Zero-based  InputPortWidth=40  IndexOptions=Index vector (port)  Indices=[1 3]  OutputSizes=1
  Subsystem6 : Subsystem
  FUS_Vision_OD_st : Outport
  wires:
  Constant/1 -> Selector/2
  OBJ_BUS/1 -> Selector9/1, Selector39/1, Selector38/1, Selector37/1, Selector36/1, Selector35/1, Selector34/1, Selector33/1, Selector32/1, Selector31/1, Selector23/1, Selector22/1, Selector21/1, Selector20/1, Selector19/1, Selector18/1, Selector17/1, Selector30/1, Selector29/1, Selector28/1, Selector27/1, Selector26/1, Selector25/1, Selector24/1, Selector16/1, Selector15/1, Selector14/1, Selector13/1, Selector12/1, Selector11/1, Selector10/1, Selector8/1, Selector7/1, Selector6/1, Selector5/1, Selector4/1, Selector3/1, Selector2/1, Selector1/1, Selector/1
  Constant1/1 -> Selector1/2
  Constant2/1 -> Selector2/2
  Constant3/1 -> Selector3/2
  Constant4/1 -> Selector4/2
  Constant5/1 -> Selector5/2
  Constant6/1 -> Selector6/2
  Constant7/1 -> Selector7/2
  Constant8/1 -> Selector8/2
  Constant9/1 -> Selector9/2
  Constant11/1 -> Selector11/2
  Constant12/1 -> Selector12/2
  Constant13/1 -> Selector13/2
  Constant14/1 -> Selector14/2
  Constant10/1 -> Selector10/2
  Constant15/1 -> Selector15/2
  Constant16/1 -> Selector16/2
  Constant17/1 -> Selector24/2
  Constant18/1 -> Selector25/2
  Constant19/1 -> Selector26/2
  Constant20/1 -> Selector27/2
  Constant21/1 -> Selector28/2
  Constant22/1 -> Selector29/2
  Constant23/1 -> Selector30/2
  Constant24/1 -> Selector17/2
  Constant25/1 -> Selector18/2
  Constant26/1 -> Selector19/2
  Constant27/1 -> Selector20/2
  Constant28/1 -> Selector21/2
  Constant29/1 -> Selector22/2
  Constant30/1 -> Selector23/2
  Constant31/1 -> Selector31/2
  Constant32/1 -> Selector32/2
  Constant33/1 -> Selector33/2
  Constant34/1 -> Selector34/2
  Constant35/1 -> Selector35/2
  Constant36/1 -> Selector36/2
  Constant37/1 -> Selector37/2
  Constant38/1 -> Selector38/2
  Constant39/1 -> Selector39/2
  Selector/1 -> Obj_1/1(EyeQ4_Obj_01)
  Selector1/1 -> Obj_2/1(EyeQ4_Obj_01)
  Obj_1/1(Obj_01_st) -> Bus Creator/1
  Obj_2/1(Obj_01_st) -> Bus Creator/2
  Bus Creator1/1 -> FUS_Vision_OD_st/1
  Obj_Frame_Info/1 -> Bus Selector/1
  Bus Selector/1 -> Data Type Conversion/1  "<SyncID>"
  Constant40/1 -> Bus Creator1/3  "Count"
  Obj_reserved1/1(reserved1) -> Bus Creator1/4  "reserved1"
  Bus Creator/1 -> Bus Creator1/5  "ObjList"
  Constant41/1 -> Bus Creator1/6  "dayNightState"
  Subsystem6/1(reserved2) -> Bus Creator1/7  "reserved2"
  Constant42/1 -> Bus Creator1/1  "timestamp"
  Data Type Conversion/1 -> Bus Creator1/2  "frameNum"
  Obj_4/1(Obj_01_st) -> Bus Creator/4
  Selector2/1 -> Obj_3/1(EyeQ4_Obj_01)
  Obj_3/1(Obj_01_st) -> Bus Creator/3
  Selector3/1 -> Obj_4/1(EyeQ4_Obj_01)
  Obj_6/1(Obj_01_st) -> Bus Creator/6
  Selector4/1 -> Obj_5/1(EyeQ4_Obj_01)
  Obj_7/1(Obj_01_st) -> Bus Creator/7
  Selector7/1 -> Obj_8/1(EyeQ4_Obj_01)
  Obj_8/1(Obj_01_st) -> Bus Creator/8
  Selector6/1 -> Obj_7/1(EyeQ4_Obj_01)
  Obj_5/1(Obj_01_st) -> Bus Creator/5
  Selector5/1 -> Obj_6/1(EyeQ4_Obj_01)
  Obj_10/1(Obj_01_st) -> Bus Creator/10
  Selector10/1 -> Obj_11/1(EyeQ4_Obj_01)
  Obj_11/1(Obj_01_st) -> Bus Creator/11
  Selector9/1 -> Obj_10/1(EyeQ4_Obj_01)
  Selector8/1 -> Obj_9/1(EyeQ4_Obj_01)
  Obj_9/1(Obj_01_st) -> Bus Creator/9
  Obj_13/1(Obj_01_st) -> Bus Creator/13
  Selector12/1 -> Obj_13/1(EyeQ4_Obj_01)
  Selector11/1 -> Obj_12/1(EyeQ4_Obj_01)
  Obj_12/1(Obj_01_st) -> Bus Creator/12
  Obj_16/1(Obj_01_st) -> Bus Creator/16
  Selector13/1 -> Obj_14/1(EyeQ4_Obj_01)
  Obj_15/1(Obj_01_st) -> Bus Creator/15
  Obj_14/1(Obj_01_st) -> Bus Creator/14
  Selector14/1 -> Obj_15/1(EyeQ4_Obj_01)
  Selector15/1 -> Obj_16/1(EyeQ4_Obj_01)
  Obj_19/1(Obj_01_st) -> Bus Creator/19
  Selector25/1 -> Obj_19/1(EyeQ4_Obj_01)
  Obj_21/1(Obj_01_st) -> Bus Creator/21
  Selector27/1 -> Obj_21/1(EyeQ4_Obj_01)
  Selector24/1 -> Obj_18/1(EyeQ4_Obj_01)
  Obj_22/1(Obj_01_st) -> Bus Creator/22
  Selector28/1 -> Obj_22/1(EyeQ4_Obj_01)
  Obj_20/1(Obj_01_st) -> Bus Creator/20
  Obj_18/1(Obj_01_st) -> Bus Creator/18
  Selector26/1 -> Obj_20/1(EyeQ4_Obj_01)
  Selector16/1 -> Obj_17/1(EyeQ4_Obj_01)
  Obj_17/1(Obj_01_st) -> Bus Creator/17
  Obj_26/1(Obj_01_st) -> Bus Creator/26
  Obj_25/1(Obj_01_st) -> Bus Creator/25
  Selector18/1 -> Obj_26/1(EyeQ4_Obj_01)
  Selector19/1 -> Obj_27/1(EyeQ4_Obj_01)
  Selector17/1 -> Obj_25/1(EyeQ4_Obj_01)
  Obj_27/1(Obj_01_st) -> Bus Creator/27
  Obj_24/1(Obj_01_st) -> Bus Creator/24
  Selector30/1 -> Obj_24/1(EyeQ4_Obj_01)
  Obj_23/1(Obj_01_st) -> Bus Creator/23
  Selector29/1 -> Obj_23/1(EyeQ4_Obj_01)
  Selector31/1 -> Obj_32/1(EyeQ4_Obj_01)
  Obj_31/1(Obj_01_st) -> Bus Creator/31
  Obj_28/1(Obj_01_st) -> Bus Creator/28
  Selector21/1 -> Obj_29/1(EyeQ4_Obj_01)
  Obj_29/1(Obj_01_st) -> Bus Creator/29
  Selector20/1 -> Obj_28/1(EyeQ4_Obj_01)
  Obj_30/1(Obj_01_st) -> Bus Creator/30
  Selector22/1 -> Obj_30/1(EyeQ4_Obj_01)
  Obj_32/1(Obj_01_st) -> Bus Creator/32
  Selector23/1 -> Obj_31/1(EyeQ4_Obj_01)
  Obj_35/1(Obj_01_st) -> Bus Creator/35
  Obj_33/1(Obj_01_st) -> Bus Creator/33
  Obj_34/1(Obj_01_st) -> Bus Creator/34
  Obj_36/1(Obj_01_st) -> Bus Creator/36
  Selector32/1 -> Obj_33/1(EyeQ4_Obj_01)
  Selector34/1 -> Obj_35/1(EyeQ4_Obj_01)
  Selector35/1 -> Obj_36/1(EyeQ4_Obj_01)
  Selector33/1 -> Obj_34/1(EyeQ4_Obj_01)
  Selector36/1 -> Obj_37/1(EyeQ4_Obj_01)
  Obj_37/1(Obj_01_st) -> Bus Creator/37
  Obj_39/1(Obj_01_st) -> Bus Creator/39
  Selector38/1 -> Obj_39/1(EyeQ4_Obj_01)
  Selector37/1 -> Obj_38/1(EyeQ4_Obj_01)
  Obj_38/1(Obj_01_st) -> Bus Creator/38
  Selector39/1 -> Obj_40/1(EyeQ4_Obj_01)
  Obj_40/1(Obj_01_st) -> Bus Creator/40

== system fusionAlg/FUSION /FUS_DataAdapter/VisionAdapter/RoadEdgeAdapter ==
  <ROADEDGE_ST> : Inport
  Bus Creator : BusCreator  Inputs=8  OutDataTypeStr=Bus: FUS_EYEQ4_ROADEDGE_DATA_ST  NonVirtualBus=on
      settings: InheritFromInputs=off
  Bus Selector1 : BusSelector  OutputSignals=RoadEdgeProtHeader,RoadEdgeProtA,RoadEdgeProtB,RoadEdgeProtC
  Constant : Constant  OutDataTypeStr=uint32
  Constant1 : Constant  Value=0  OutDataTypeStr=uint32
  Constant2 : Constant  Value=0  OutDataTypeStr=uint32
  RoadEdgeProtAAdapter : Subsystem
  RoadEdgeProtBAdapter : Subsystem
  RoadEdgeProtCAdapter : Subsystem
  RoadEdgeProtHeaderAdapter : Subsystem
  constant : Constant  Value=1012  OutDataTypeStr=double
  FUS_RoadEdge_st : Outport  OutDataTypeStr=Bus: FUS_EYEQ4_ROADEDGE_DATA_ST
  wires:
  Bus Creator/1 -> FUS_RoadEdge_st/1
  <ROADEDGE_ST>/1 -> Bus Selector1/1
  constant/1 -> Bus Creator/1
  Constant/1 -> Bus Creator/2
  Bus Selector1/1 -> RoadEdgeProtHeaderAdapter/1(<RoadEdgeProtHeader>)  "<RoadEdgeProtHeader>"
  RoadEdgeProtHeaderAdapter/1(RoadEdgeProtHeader) -> Bus Creator/3  "ProtHeader"
  Bus Selector1/2 -> RoadEdgeProtAAdapter/1(<RoadEdgeProtA>)  "<RoadEdgeProtA>"
  RoadEdgeProtAAdapter/1(RoadEdgeProtA) -> Bus Creator/4  "ProtA"
  Bus Selector1/3 -> RoadEdgeProtBAdapter/1(<RoadEdgeProtB>)  "<RoadEdgeProtB>"
  RoadEdgeProtBAdapter/1(RoadEdgeProtB) -> Bus Creator/5  "ProtB"
  Bus Selector1/4 -> RoadEdgeProtCAdapter/1(<RoadEdgeProtC>)  "<RoadEdgeProtC>"
  RoadEdgeProtCAdapter/1(RoadEdgeProtC) -> Bus Creator/6  "ProtC"
  Constant1/1 -> Bus Creator/7
  Constant2/1 -> Bus Creator/8

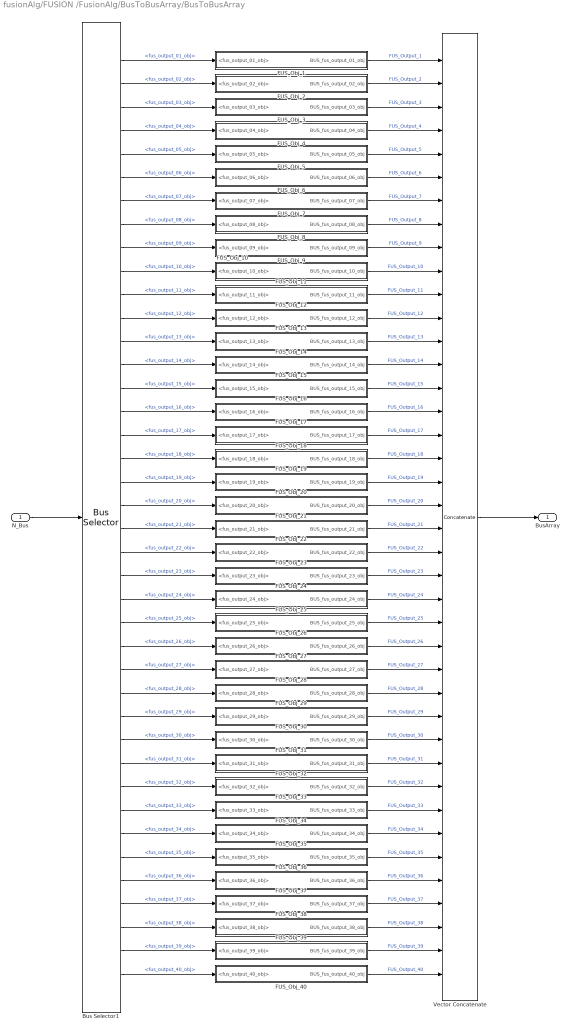
== system fusionAlg/FUSION /FusionAlg/BusToBusArray/BusToBusArray ==
  N_Bus : Inport
  Bus Selector1 : BusSelector  OutputSignals=fus_output_01_obj,fus_output_02_obj,fus_output_03_obj,fus_output_04_obj,fus_output_05_obj,fus_output_06_obj,fus_output_07_obj,fus_output_08_obj,fus_output_09_obj,fus_output_10_obj,fus_output_11_obj,fus_output_12_obj,fus_output_13_obj,fus_output_14_obj,fus_output_15_obj,fus_output_16_obj,fus_output_17_obj,fus_output_18_obj,fus_output_19_obj,fus_output_20_obj,fus_output_21_obj,fus_output_22_obj,fus_output_23_obj,fus_output_24_obj,fus_output_25_obj,fus_output_26_obj,fus_output_27_obj,fus_output_28_obj,fus_output_29_obj,fus_output_30_obj,fus_output_31_obj,fus_output_32_obj,fus_output_33_obj,fus_output_34_obj,fus_output_35_obj,fus_output_36_obj,fus_output_37_obj,fus_output_38_obj,fus_output_39_obj,fus_output_40_obj
  FUS_Obj_1 : Subsystem
  FUS_Obj_10 : Subsystem
  FUS_Obj_11 : Subsystem
  FUS_Obj_12 : Subsystem
  FUS_Obj_13 : Subsystem
  FUS_Obj_14 : Subsystem
  FUS_Obj_15 : Subsystem
  FUS_Obj_16 : Subsystem
  FUS_Obj_17 : Subsystem
  FUS_Obj_18 : Subsystem
  FUS_Obj_19 : Subsystem
  FUS_Obj_2 : Subsystem
  FUS_Obj_20 : Subsystem
  FUS_Obj_21 : Subsystem
  FUS_Obj_22 : Subsystem
  FUS_Obj_23 : Subsystem
  FUS_Obj_24 : Subsystem
  FUS_Obj_25 : Subsystem
  FUS_Obj_26 : Subsystem
  FUS_Obj_27 : Subsystem
  FUS_Obj_28 : Subsystem
  FUS_Obj_29 : Subsystem
  FUS_Obj_3 : Subsystem
  FUS_Obj_30 : Subsystem
  FUS_Obj_31 : Subsystem
  FUS_Obj_32 : Subsystem
  FUS_Obj_33 : Subsystem
  FUS_Obj_34 : Subsystem
  FUS_Obj_35 : Subsystem
  FUS_Obj_36 : Subsystem
  FUS_Obj_37 : Subsystem
  FUS_Obj_38 : Subsystem
  FUS_Obj_39 : Subsystem
  FUS_Obj_4 : Subsystem
  FUS_Obj_40 : Subsystem
  FUS_Obj_5 : Subsystem
  FUS_Obj_6 : Subsystem
  FUS_Obj_7 : Subsystem
  FUS_Obj_8 : Subsystem
  FUS_Obj_9 : Subsystem
  Vector Concatenate : Concatenate  NumInputs=40
  BusArray : Outport
  wires:
  N_Bus/1 -> Bus Selector1/1
  Vector Concatenate/1 -> BusArray/1
  Bus Selector1/1 -> FUS_Obj_1/1(<fus_output_01_obj>)  "<fus_output_01_obj>"
  Bus Selector1/2 -> FUS_Obj_2/1(<fus_output_02_obj>)  "<fus_output_02_obj>"
  FUS_Obj_2/1(BUS_fus_output_02_obj) -> Vector Concatenate/2  "FUS_Output_2"
  Bus Selector1/3 -> FUS_Obj_3/1(<fus_output_03_obj>)  "<fus_output_03_obj>"
  Bus Selector1/4 -> FUS_Obj_4/1(<fus_output_04_obj>)  "<fus_output_04_obj>"
  FUS_Obj_1/1(BUS_fus_output_01_obj) -> Vector Concatenate/1  "FUS_Output_1"
  FUS_Obj_3/1(BUS_fus_output_03_obj) -> Vector Concatenate/3  "FUS_Output_3"
  FUS_Obj_4/1(BUS_fus_output_04_obj) -> Vector Concatenate/4  "FUS_Output_4"
  FUS_Obj_5/1(BUS_fus_output_05_obj) -> Vector Concatenate/5  "FUS_Output_5"
  Bus Selector1/10 -> FUS_Obj_10/1(<fus_output_10_obj>)  "<fus_output_10_obj>"
  FUS_Obj_13/1(BUS_fus_output_13_obj) -> Vector Concatenate/13  "FUS_Output_13"
  FUS_Obj_9/1(BUS_fus_output_09_obj) -> Vector Concatenate/9  "FUS_Output_9"
  FUS_Obj_12/1(BUS_fus_output_12_obj) -> Vector Concatenate/12  "FUS_Output_12"
  Bus Selector1/9 -> FUS_Obj_9/1(<fus_output_09_obj>)  "<fus_output_09_obj>"
  FUS_Obj_11/1(BUS_fus_output_11_obj) -> Vector Concatenate/11  "FUS_Output_11"
  Bus Selector1/11 -> FUS_Obj_11/1(<fus_output_11_obj>)  "<fus_output_11_obj>"
  FUS_Obj_10/1(BUS_fus_output_10_obj) -> Vector Concatenate/10  "FUS_Output_10"
  Bus Selector1/12 -> FUS_Obj_12/1(<fus_output_12_obj>)  "<fus_output_12_obj>"
  FUS_Obj_6/1(BUS_fus_output_06_obj) -> Vector Concatenate/6  "FUS_Output_6"
  FUS_Obj_7/1(BUS_fus_output_07_obj) -> Vector Concatenate/7  "FUS_Output_7"
  FUS_Obj_8/1(BUS_fus_output_08_obj) -> Vector Concatenate/8  "FUS_Output_8"
  Bus Selector1/5 -> FUS_Obj_5/1(<fus_output_05_obj>)  "<fus_output_05_obj>"
  Bus Selector1/6 -> FUS_Obj_6/1(<fus_output_06_obj>)  "<fus_output_06_obj>"
  Bus Selector1/7 -> FUS_Obj_7/1(<fus_output_07_obj>)  "<fus_output_07_obj>"
  Bus Selector1/8 -> FUS_Obj_8/1(<fus_output_08_obj>)  "<fus_output_08_obj>"
  Bus Selector1/13 -> FUS_Obj_13/1(<fus_output_13_obj>)  "<fus_output_13_obj>"
  Bus Selector1/14 -> FUS_Obj_14/1(<fus_output_14_obj>)  "<fus_output_14_obj>"
  Bus Selector1/15 -> FUS_Obj_15/1(<fus_output_15_obj>)  "<fus_output_15_obj>"
  Bus Selector1/16 -> FUS_Obj_16/1(<fus_output_16_obj>)  "<fus_output_16_obj>"
  FUS_Obj_14/1(BUS_fus_output_14_obj) -> Vector Concatenate/14  "FUS_Output_14"
  FUS_Obj_15/1(BUS_fus_output_15_obj) -> Vector Concatenate/15  "FUS_Output_15"
  FUS_Obj_16/1(BUS_fus_output_16_obj) -> Vector Concatenate/16  "FUS_Output_16"
  Bus Selector1/19 -> FUS_Obj_19/1(<fus_output_19_obj>)  "<fus_output_19_obj>"
  FUS_Obj_27/1(BUS_fus_output_27_obj) -> Vector Concatenate/27  "FUS_Output_27"
  FUS_Obj_19/1(BUS_fus_output_19_obj) -> Vector Concatenate/19  "FUS_Output_19"
  Bus Selector1/18 -> FUS_Obj_18/1(<fus_output_18_obj>)  "<fus_output_18_obj>"
  Bus Selector1/22 -> FUS_Obj_22/1(<fus_output_22_obj>)  "<fus_output_22_obj>"
  Bus Selector1/25 -> FUS_Obj_25/1(<fus_output_25_obj>)  "<fus_output_25_obj>"
  FUS_Obj_18/1(BUS_fus_output_18_obj) -> Vector Concatenate/18  "FUS_Output_18"
  FUS_Obj_29/1(BUS_fus_output_29_obj) -> Vector Concatenate/29  "FUS_Output_29"
  FUS_Obj_23/1(BUS_fus_output_23_obj) -> Vector Concatenate/23  "FUS_Output_23"
  FUS_Obj_25/1(BUS_fus_output_25_obj) -> Vector Concatenate/25  "FUS_Output_25"
  FUS_Obj_20/1(BUS_fus_output_20_obj) -> Vector Concatenate/20  "FUS_Output_20"
  FUS_Obj_24/1(BUS_fus_output_24_obj) -> Vector Concatenate/24  "FUS_Output_24"
  Bus Selector1/23 -> FUS_Obj_23/1(<fus_output_23_obj>)  "<fus_output_23_obj>"
  FUS_Obj_22/1(BUS_fus_output_22_obj) -> Vector Concatenate/22  "FUS_Output_22"
  FUS_Obj_26/1(BUS_fus_output_26_obj) -> Vector Concatenate/26  "FUS_Output_26"
  Bus Selector1/21 -> FUS_Obj_21/1(<fus_output_21_obj>)  "<fus_output_21_obj>"
  Bus Selector1/28 -> FUS_Obj_28/1(<fus_output_28_obj>)  "<fus_output_28_obj>"
  Bus Selector1/20 -> FUS_Obj_20/1(<fus_output_20_obj>)  "<fus_output_20_obj>"
  Bus Selector1/29 -> FUS_Obj_29/1(<fus_output_29_obj>)  "<fus_output_29_obj>"
  FUS_Obj_17/1(BUS_fus_output_17_obj) -> Vector Concatenate/17  "FUS_Output_17"
  Bus Selector1/24 -> FUS_Obj_24/1(<fus_output_24_obj>)  "<fus_output_24_obj>"
  FUS_Obj_21/1(BUS_fus_output_21_obj) -> Vector Concatenate/21  "FUS_Output_21"
  FUS_Obj_28/1(BUS_fus_output_28_obj) -> Vector Concatenate/28  "FUS_Output_28"
  Bus Selector1/27 -> FUS_Obj_27/1(<fus_output_27_obj>)  "<fus_output_27_obj>"
  Bus Selector1/17 -> FUS_Obj_17/1(<fus_output_17_obj>)  "<fus_output_17_obj>"
  Bus Selector1/26 -> FUS_Obj_26/1(<fus_output_26_obj>)  "<fus_output_26_obj>"
  FUS_Obj_35/1(BUS_fus_output_35_obj) -> Vector Concatenate/35  "FUS_Output_35"
  FUS_Obj_40/1(BUS_fus_output_40_obj) -> Vector Concatenate/40  "FUS_Output_40"
  FUS_Obj_34/1(BUS_fus_output_34_obj) -> Vector Concatenate/34  "FUS_Output_34"
  FUS_Obj_39/1(BUS_fus_output_39_obj) -> Vector Concatenate/39  "FUS_Output_39"
  FUS_Obj_38/1(BUS_fus_output_38_obj) -> Vector Concatenate/38  "FUS_Output_38"
  FUS_Obj_32/1(BUS_fus_output_32_obj) -> Vector Concatenate/32  "FUS_Output_32"
  FUS_Obj_31/1(BUS_fus_output_31_obj) -> Vector Concatenate/31  "FUS_Output_31"
  FUS_Obj_36/1(BUS_fus_output_36_obj) -> Vector Concatenate/36  "FUS_Output_36"
  FUS_Obj_37/1(BUS_fus_output_37_obj) -> Vector Concatenate/37  "FUS_Output_37"
  FUS_Obj_30/1(BUS_fus_output_30_obj) -> Vector Concatenate/30  "FUS_Output_30"
  Bus Selector1/38 -> FUS_Obj_38/1(<fus_output_38_obj>)  "<fus_output_38_obj>"
  Bus Selector1/34 -> FUS_Obj_34/1(<fus_output_34_obj>)  "<fus_output_34_obj>"
  Bus Selector1/36 -> FUS_Obj_36/1(<fus_output_36_obj>)  "<fus_output_36_obj>"
  Bus Selector1/39 -> FUS_Obj_39/1(<fus_output_39_obj>)  "<fus_output_39_obj>"
  Bus Selector1/40 -> FUS_Obj_40/1(<fus_output_40_obj>)  "<fus_output_40_obj>"
  Bus Selector1/37 -> FUS_Obj_37/1(<fus_output_37_obj>)  "<fus_output_37_obj>"
  FUS_Obj_33/1(BUS_fus_output_33_obj) -> Vector Concatenate/33  "FUS_Output_33"
  Bus Selector1/32 -> FUS_Obj_32/1(<fus_output_32_obj>)  "<fus_output_32_obj>"
  Bus Selector1/31 -> FUS_Obj_31/1(<fus_output_31_obj>)  "<fus_output_31_obj>"
  Bus Selector1/33 -> FUS_Obj_33/1(<fus_output_33_obj>)  "<fus_output_33_obj>"
  Bus Selector1/35 -> FUS_Obj_35/1(<fus_output_35_obj>)  "<fus_output_35_obj>"
  Bus Selector1/30 -> FUS_Obj_30/1(<fus_output_30_obj>)  "<fus_output_30_obj>"

== system fusionAlg/RTI Data/RTI Data Store/RTI Data Store/RTI Data Store ==
  RTI Data Store : Subsystem  mask(RTI_DATA_STORE){}
      mask help:
      | RTI Data Store Block. This block is used by RTI to store internal model dependent data. Deleting this block will result in data loss.
      |
      | NEVER DELETE, COPY, OR MODIFY THIS BLOCK!
      mask Help:
      | RTI Data Store Block. This block is used by RTI to store internal model dependent data. Deleting this block will result in data loss.
      | 
      | NEVER DELETE, COPY, OR MODIFY THIS BLOCK!
      mask Display: text(0.5, 0.5, ' ', 'HorizontalAlignment', 'center');
